simulink model "FOPTD_Relay_Feedback_sim"  (R2014a)
settings: Solver=ode45  StartTime=0.0  StopTime=100.0  RelTol=1e-3
settings Model: Creator=38128  LastModifiedBy=38128

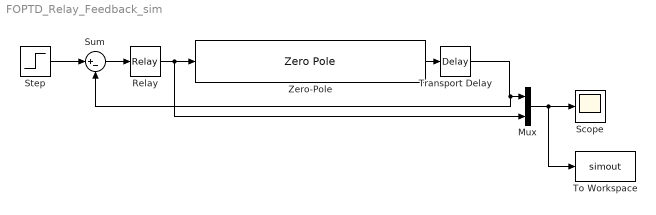
== system FOPTD_Relay_Feedback_sim ==
  Mux : Mux  Inputs=2
  Relay : Relay  OnSwitchValue=0  OffSwitchValue=0  OffOutputValue=-1
  Scope : Scope
      settings: TimeRange=100
  Step : Step  Time=65  SampleTime=0
  Sum : Sum  Inputs=|+-
  To Workspace : ToWorkspace  VariableName=simout  SaveFormat=Timeseries  SampleTime=-1
  Transport Delay : TransportDelay  DelayTime=2.5
  Zero-Pole : ZeroPole  Zeros=[-3.5]  Poles=[-1 -1 -1 -2 -2 -2 -5]
  wires:
  Step/1 -> Sum/1
  Zero-Pole/1 -> Transport Delay/1
  Transport Delay/1 -> Sum/2, Mux/1
  Mux/1 -> To Workspace/1, Scope/1
  Sum/1 -> Relay/1
  Relay/1 -> Mux/2, Zero-Pole/1
